simulink model "gm_HDLRx_vs"  (R2024a)
settings: Solver=FixedStepDiscrete  StartTime=0.0  StopTime=stopTime  RelTol=1e-3
undefined symbols (not defined in the file or in its folder): channelBitsPerSubcarrier, channelCyclicPrefixLen, channelOFDMSamples, channelScramblerInit, clk, clk_enable, decimatorDelay, decimatorFilter, fPHY, fs, headerBitsPerFec, headerBitsPerSubcarrier, headerCyclicPrefixLen, headerOFDMSamples, headerScramblerInit, lowerbound, N, numDataCarriers, payloadBitsPerFec, payloadScramblerInit, preambleBitsPerSubcarrier, preambleCyclicPrefixLen, preambleFirstPartOFDMSamples, preambleScramblerInit, preambleSecondPartOFDMSamples, QAM, reset_x, upperbound
libraries: hdlsllib x133, hdlmdlgenlib x132, simulink x8, whdlutilities x8, whdlmod x4, dspsrcs4 x2, whdledac x2, commhdlcrc x1, dsphdlfiltering2 x1, dsphdlsigops2 x1, vivadosimlib x1, HDL_ieee_8021513 x1
(part 4 of 4)

== matlab function gm_HDLRx_vs/full_rx/rx_demodulator_full/ofdm_separator/Real Divide HDL Optimized/ForEach - Real Divide_instance1/Normalize denominator/positiveRealNormalizer/embreciprocals_c3_szUwl4UaRWSwHB6ziXbSTrD_positiveRealNormalize ==
  settings: fimath=hdlfimath
  data: u input; x output; validIn input; e output; isNegative output; validOut output
function [x, e, isNegative, validOut] = realNormalizer(u, validIn)
    %realNormalizer Normalize real values.
    % Given real scalar u ~= 0, this block produces x such that
    %    1 <= x < 2,
    % e such that
    %    x = (2^e)*|u|,
    % and isNegative = u<0.
    %
    %   When u = 0 and u is fixed-point or scaled-double, then x = 0 and
    %   e = (2^nextpow2(x.WordLength)) - x.WordLength - x.FractionLength.
    %
    %   When u = 0 and u is floating-point, then x = 0 and e = 1.
    
    %   Copyright 2019 The MathWorks, Inc.
    %#codegen
    
    % This function only works on scalars.
    % Only operate on the real part
    fixed.internal.reciprocal.validateNormalizerInputs(u, validIn);
    % Normalize in unsigned type.
    [x_normalized, n_normalized, isNegative, validOut] = normalize(real(u), validIn);
    % Cast the output to signed if the input was signed.
    x = fixed.internal.reciprocal.castToInputSignedness(x_normalized,u);
    % Convert the normalized shift value based on the data type of the
    % input U so that the output of the normalizer X is in real-world
    % scale and X = (2^N)*U.
    e = fi(int32(0));
    e(:) = fixed.internal.reciprocal.normalizedShiftToRealWorldValueShift(n_normalized,u);
end

function [x_normalized, e_normalized, isNegative, validOut] = normalize(u, validIn)
    [u, isNegative] = fixed.reciprocal.pipelined.makeRealScalarPositive(u);
    if isfi(u) && isfixed(u)
        % Normalize fixed-point values
        [x_normalized, e_normalized, isNegative, validOut] = normalizeFixedpoint(u, isNegative, validIn);
    else
        % Normalize floating-point or scaled-double
        [x_normalized, e_normalized, validOut] = fixed.internal.reciprocal.normalizePositiveFloatOrScaledDouble(u, validIn);
    end
end

function [u_normalized, e_normalized, isNegativeOut, validOut] = normalizeFixedpoint(u, isNegative, validIn)
    % Normalize fixed-point values.
    persistent validReg
    persistent tReg
    persistent xReg
    persistent isNegativeReg
    % For fixed-point types, the normalization uses a binary search of
    % length log2 of the word length of the input.
    number_of_stages = coder.const(nextpow2(u.WordLength));
    
    if isempty(validReg)
        validReg = false(number_of_stages+1,1);
        tReg = zeros(number_of_stages+1,1,'like',fi(0,0,max(number_of_stages,1),0));
        xReg = zeros(number_of_stages+1,1,'like',fi([],0,u.WordLength,0));
        isNegativeReg = false(number_of_stages+1,1);
    end
    
    [u_normalized, e_normalized,validOut,...
        validReg, tReg,xReg...  % Persistent
        ] = fixed.internal.reciprocal.normalizePositiveFixedPoint(u, validIn, number_of_stages, ...
        validReg, tReg,xReg...  % Persistent
        );
    % Assign outputs from states
    isNegativeOut = isNegativeReg(end);
    
    % Update isNegative states
    coder.unroll;
    for k = number_of_stages:-1:1
        isNegativeReg(k+1) = isNegativeReg(k);
    end
    isNegativeReg(1) = isNegative;
end

== matlab function gm_HDLRx_vs/full_rx/rx_demodulator_full/ofdm_separator/Real Divide HDL Optimized/ForEach - Real Divide_instance1/Normalize numerator/positiveRealNormalizer/embreciprocals_c3_s14mscxAahtiBqnXaktE2fE_positiveRealNormalize ==
  settings: fimath=hdlfimath
  data: u input; x output; validIn input; e output; isNegative output; validOut output
function [x, e, isNegative, validOut] = realNormalizer(u, validIn)
    %realNormalizer Normalize real values.
    % Given real scalar u ~= 0, this block produces x such that
    %    1 <= x < 2,
    % e such that
    %    x = (2^e)*|u|,
    % and isNegative = u<0.
    %
    %   When u = 0 and u is fixed-point or scaled-double, then x = 0 and
    %   e = (2^nextpow2(x.WordLength)) - x.WordLength - x.FractionLength.
    %
    %   When u = 0 and u is floating-point, then x = 0 and e = 1.
    
    %   Copyright 2019 The MathWorks, Inc.
    %#codegen
    
    % This function only works on scalars.
    % Only operate on the real part
    fixed.internal.reciprocal.validateNormalizerInputs(u, validIn);
    % Normalize in unsigned type.
    [x_normalized, n_normalized, isNegative, validOut] = normalize(real(u), validIn);
    % Cast the output to signed if the input was signed.
    x = fixed.internal.reciprocal.castToInputSignedness(x_normalized,u);
    % Convert the normalized shift value based on the data type of the
    % input U so that the output of the normalizer X is in real-world
    % scale and X = (2^N)*U.
    e = fi(int32(0));
    e(:) = fixed.internal.reciprocal.normalizedShiftToRealWorldValueShift(n_normalized,u);
end

function [x_normalized, e_normalized, isNegative, validOut] = normalize(u, validIn)
    [u, isNegative] = fixed.reciprocal.pipelined.makeRealScalarPositive(u);
    if isfi(u) && isfixed(u)
        % Normalize fixed-point values
        [x_normalized, e_normalized, isNegative, validOut] = normalizeFixedpoint(u, isNegative, validIn);
    else
        % Normalize floating-point or scaled-double
        [x_normalized, e_normalized, validOut] = fixed.internal.reciprocal.normalizePositiveFloatOrScaledDouble(u, validIn);
    end
end

function [u_normalized, e_normalized, isNegativeOut, validOut] = normalizeFixedpoint(u, isNegative, validIn)
    % Normalize fixed-point values.
    persistent validReg
    persistent tReg
    persistent xReg
    persistent isNegativeReg
    % For fixed-point types, the normalization uses a binary search of
    % length log2 of the word length of the input.
    number_of_stages = coder.const(nextpow2(u.WordLength));
    
    if isempty(validReg)
        validReg = false(number_of_stages+1,1);
        tReg = zeros(number_of_stages+1,1,'like',fi(0,0,max(number_of_stages,1),0));
        xReg = zeros(number_of_stages+1,1,'like',fi([],0,u.WordLength,0));
        isNegativeReg = false(number_of_stages+1,1);
    end
    
    [u_normalized, e_normalized,validOut,...
        validReg, tReg,xReg...  % Persistent
        ] = fixed.internal.reciprocal.normalizePositiveFixedPoint(u, validIn, number_of_stages, ...
        validReg, tReg,xReg...  % Persistent
        );
    % Assign outputs from states
    isNegativeOut = isNegativeReg(end);
    
    % Update isNegative states
    coder.unroll;
    for k = number_of_stages:-1:1
        isNegativeReg(k+1) = isNegativeReg(k);
    end
    isNegativeReg(1) = isNegative;
end

== matlab function gm_HDLRx_vs/full_rx/rx_demodulator_full/ofdm_separator/Real Divide HDL Optimized/ForEach - Real Divide_instance1/Upcast Wordlength/slutils_c2_Upcast_Wordlength ==
  data: x input; u output; y input; v output
function [u, v] = upcastWordlength(x, y)

% Copyright 2019 The MathWorks, Inc.

%#codegen

[u, v] = fixed.internal.type.upcastWordlength(x,y);

end

== matlab function gm_HDLRx_vs/full_rx/rx_demodulator_full/ofdm_separator/Real Divide HDL Optimized/Reshape to original size/embreciprocals_c11_Reshape_to_original_size ==
  data: y input; u input; z output
function z = reshape_to_original_size(y,u)
    z = reshape(y,size(u));
end

== matlab function gm_HDLRx_vs/full_rx/rx_demodulator_full/ofdm_separator/Real Divide HDL Optimized/ForEach - Real Divide_instance1/MATLAB Function/embreciprocals_c13_MATLAB_Function ==
  settings: fimath=hdlfimath
  data: num input; num_out output; t_num input; t_num_out output
function [num_out, t_num_out] = fcn(num, t_num)

num_out = bitsra(num,1);
t_num_out = t_num - 1;

end

== matlab function gm_HDLRx_vs/full_rx/rx_demodulator_full/ofdm_separator/Real Divide HDL Optimized/Verify divide sizes/embreciprocals_c19_Verify_divide_sizes ==
  data: denominator input; den output; numerator input; num output
function [den,num] = verify_size(denominator,numerator)
   % Verify that the dimensions of the input arrays match, and then reshape
   % them.
   coder.internal.assert(numel(denominator)==numel(numerator),...
       'fixed:emblib:DivideDimensionsShouldMatch',...
       'Real Divide HDL Optimized');
   num = reshape(numerator,1,numel(numerator));
   den = reshape(denominator,1,numel(denominator));
end

== matlab function gm_HDLRx_vs/full_rx/rx_demodulator_full/ofdm_separator/Real Divide HDL Optimized/ForEach - Real Divide_instance1/Divide real numerator by denominator/normalizedCORDICDivide/embreciprocals_c21_normalizedCORDICDivide ==
  settings: fimath=hdlfimath
  data: num input; den input; tNum input; tDen input; isNumNegative input; isDenNegative input; y output; t output; isDenZeroOut output; validIn input; validOut output
function [y, t, isDenZeroOut, validOut] = normalizedCORDICDivide(num, den, tNum, tDen, isNumNegative, isDenNegative, validIn)
    %   Copyright 2020 The MathWorks, Inc.
    %#codegen
    fixed.internal.reciprocal.validateReciprocalInputs(num, validIn);
    if isfi(num) && isscaledtype(num)
        isDenZero = den==0;
        isNumZero = num==0;
        % CORDIC divide for fixed-point and scaled-double types
        [y,t,isNegative,isNumZeroOut, isDenZeroOut,validOut] = fixedpointDivide(den,num,tDen-tNum,isNumNegative ~= isDenNegative, isNumZero, isDenZero,validIn);
    else
        % y = num/den for builtin types.
        y = num./den;
        t = tDen - tNum;
        isNegative = isNumNegative ~= isDenNegative;
        validOut = validIn;
        isDenZeroOut = false;
        isNumZeroOut = false;
    end
    if isNumZeroOut
        % Negate with saturate so the most negative value doesn't overflow.
        F = fimath('OverflowAction', 'Saturate');
        y(:) = setfimath(0,F);
    else
        if isNegative
            % Negate with saturate so the most negative value doesn't overflow.
            F = fimath('OverflowAction', 'Saturate');
            y(:) = -setfimath(y,F);
        end
    end
end

function [division, t, isNegativeOut, isNumZeroOut, isDenZeroOut, validOut] = fixedpointDivide(x,y,t_in,isNegative,isNumZero,isDenZero,validIn)
    T = fixed.cordic.linear.positiveReciprocalTypes(x);
    maximumShiftValue = coder.const(fixed.cordic.maximumShiftValue(T.data));
    % Register variables for the CORDIC Divide Kernel
    persistent xReg yReg zReg validReg tReg isNegativeReg isNumZeroReg isDenZeroReg
    if isempty(xReg)
        xReg = zeros(maximumShiftValue+2,1,'like',T.data);
        yReg = zeros(maximumShiftValue+2,1,'like',T.data);
        zReg = zeros(maximumShiftValue+2,1,'like',T.data);
        validReg = zeros(maximumShiftValue+2,1,'like',validIn);
        tReg = zeros(maximumShiftValue+2,1,'like',t_in);
        isNegativeReg = false(maximumShiftValue+2,1);
        isDenZeroReg = false(maximumShiftValue+2,1);
        isNumZeroReg = false(maximumShiftValue+2,1);
    end
    % CORDIC Divide Kernel
    [division,t,validOut,...
        xReg,yReg,zReg,validReg,tReg... % Persistent variables
        ] = fixed.internal.reciprocal.cordicDivideKernel(x,y,t_in,validIn,...
        xReg,yReg,zReg,validReg,tReg... % Persistent variables
        );
    
    % Assign outputs from states
    isNegativeOut = isNegativeReg(end);
    isNumZeroOut = isNumZeroReg(end);
    isDenZeroOut = isDenZeroReg(end);
    % Update isNegative states
    coder.unroll
    for k = maximumShiftValue+1:-1:1
        isNegativeReg(k+1) = isNegativeReg(k);
        isNumZeroReg(k+1) = isNumZeroReg(k);
        isDenZeroReg(k+1) = isDenZeroReg(k);
    end
    isNegativeReg(1) = isNegative;
    isNumZeroReg(1) = isNumZero;
    isDenZeroReg(1) = isDenZero;
end
